simulink model "npc_system"  (R2022a)
settings: Solver=FixedStepDiscrete  StartTime=0.0  StopTime=1  FixedStep=step_size  RelTol=1e-3  EnableMultiTasking=on
values from neighbouring files (symbols this model uses):
  P = 11000.0    [param.sldd]
  step_size = 1.0E-7    [param.sldd]
  Tsw = 1.5E-5    [param.sldd]
undefined symbols (not defined in the file or in its folder): D1, DiscIntNeverNeededParam
libraries: simulink x14, eeGeneralControl x3, simulink_extras x1, spsEdgeDetectorLib x1, spsSampleandHoldLib x1
settings Model: DataDictionary=param.sldd  ExtModeTrigDuration=8  Creator=sgcesuser3  LastModifiedBy=sgcesuser3
settings SolverCC: AlgebraicLoopSolver=TrustRegion  AutoInsertRateTranBlk=on
settings DataIOCC: SaveOutput=off  SignalLogging=off  DSMLogging=off  SaveTime=off  ReturnWorkspaceOutputs=off
settings OptimizationCC: EnhancedBackFolding=on  PassReuseOutputArgsAs=Individual arguments  MaxStackSize=1024  OptimizeBlockOrder=speed  DifferentSizesBufferReuse=on  OptimizationCustomize=off  EfficientTunableParamExpr=on
settings DebuggingCC: ParameterTunabilityLossMsg=error  UnconnectedInputMsg=warning  UnconnectedOutputMsg=warning  UnconnectedLineMsg=warning  SFMachineParentedDataDiag=warning
settings HardwareCC: ProdBitPerChar=16  ProdBitPerInt=16  ProdBitPerPointer=32  ProdBitPerSizeT=32  ProdBitPerPtrDiffT=32  ProdLargestAtomicInteger=Integer  ProdLargestAtomicFloat=None  ProdWordSize=16  ProdLongLongMode=on  ProdHWDeviceType=Texas Instruments->C2000
settings ModelReferenceCC: PropagateSignalLabelsOutOfModel=off
settings SFSimCC: MATLABDynamicMemAlloc=off
settings RTWCC: SystemTargetFile=ert.tlc  HardwareBoard=TI Delfino F2837xS  TemplateMakefile=ert_default_tmf  Toolchain=Texas Instruments Code Composer Studio (C2000)  DLArmComputeVersion=19.05
settings CodeAppCC: ForceParamTrailComments=on  IgnoreCustomStorageClasses=off  OperatorAnnotations=on  SimulinkDataObjDesc=on  SFDataObjDesc=on  InsertBlockDesc=on
settings ERTTargetCC: CodeReplacementLibrary=TI C28x  ExtModeTransport=4  ExtModeStaticAlloc=on  ExtModeStaticAllocSize=5000  ExtModeMexFile=ext_xcp  ExtModeIntrfLevel=Level2 - Open

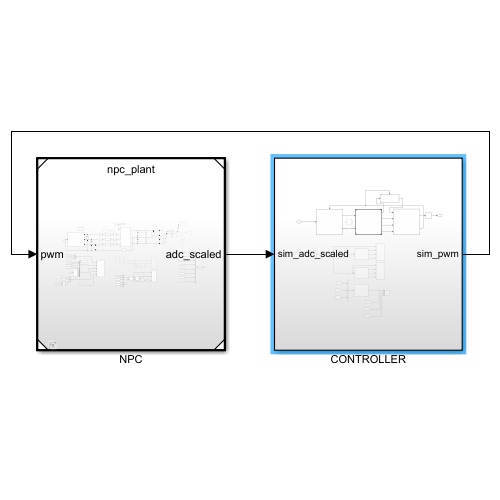
[thumbnail: Simulink's stored preview of the top-level diagram]
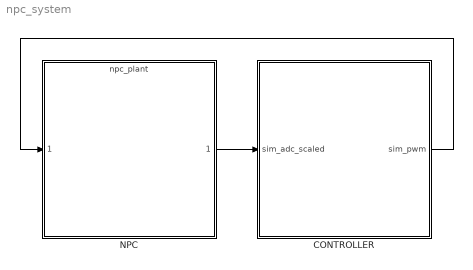
== system npc_system ==
  CONTROLLER : Subsystem
  NPC : ModelReference  ModelNameDialog=npc_plant.slx  SimulationMode=Normal  ModelReferenceVersion=4.130
  wires:
  CONTROLLER/1(sim_pwm) -> NPC/1
  NPC/1 -> CONTROLLER/1(sim_adc_scaled)

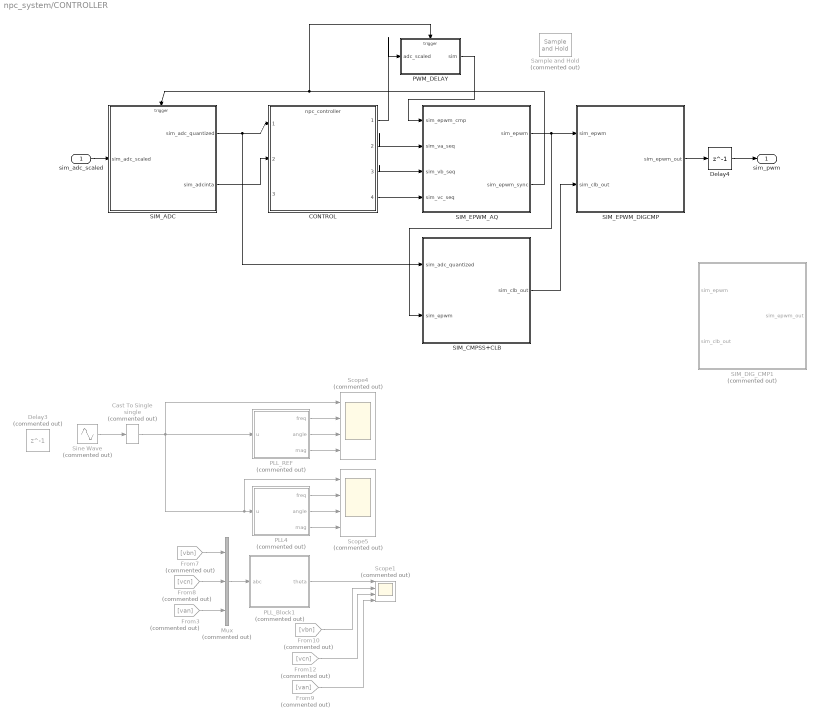
== system npc_system/CONTROLLER ==
  sim_adc_scaled : Inport
  CONTROL : ModelReference  ModelNameDialog=npc_controller.slx  SimulationMode=Normal  ScheduleRates=on  ModelEventPortInfo=P:D1[-2][0][0]  ModelReferenceVersion=4.1730
  Cast To Single : DataTypeConversion  Commented=on  OutDataTypeStr=single  SaturateOnIntegerOverflow=off  RndMeth=Floor
  Delay3 : Delay  Commented=on  DelayLength=1  InitialCondition=0
  Delay4 : Delay  DelayLength=1  InitialCondition=0
  From10 : From  Commented=on  GotoTag=vbn
  From12 : From  Commented=on  GotoTag=vcn
  From3 : From  Commented=on  GotoTag=van
  From7 : From  Commented=on  GotoTag=vbn
  From8 : From  Commented=on  GotoTag=vcn
  From9 : From  Commented=on  GotoTag=van
  Mux : Mux  Commented=on  Inputs=3
  PLL4 : Subsystem  Commented=on
  PLL_Block1 : Subsystem  Commented=on  TreatAsAtomicUnit=on
      settings: RTWFcnNameOpts=Use subsystem name
  PLL_REF : Subsystem  Commented=on
  PWM_DELAY : Subsystem  TreatAsAtomicUnit=on
  SIM_ADC : Subsystem  TreatAsAtomicUnit=on
  SIM_CMPSS+CLB : Subsystem
  SIM_DIG_CMP1 : Subsystem  Commented=on
  SIM_EPWM_AQ : Subsystem
  SIM_EPWM_DIGCMP : Subsystem
  Sample and Hold : spsSampleandHoldLib/Sample and Hold  Commented=on  ic=0  Ts=0
      settings: SourceProductBaseCode=PS
  Scope1 : Scope  Commented=on  NumInputPorts=4
  Scope4 : Scope  Commented=on  NumInputPorts=4
  Scope5 : Scope  Commented=on  NumInputPorts=4
  Sine Wave : Sin  Commented=on  Amplitude=220  Bias=100  Frequency=50*6.28
  sim_pwm : Outport
  wires:
  SIM_EPWM_AQ/2(sim_epwm_sync) -> PWM_DELAY/Trigger, SIM_ADC/Trigger
  SIM_ADC/2(sim_adcinta) -> CONTROL/2
  SIM_ADC/1(sim_adc_quantized) -> SIM_CMPSS+CLB/1(sim_adc_quantized), CONTROL/1
  PWM_DELAY/1(sim) -> SIM_EPWM_AQ/1(sim_epwm_cmp)
  CONTROL/2 -> SIM_EPWM_AQ/2(sim_va_seq)
  CONTROL/3 -> SIM_EPWM_AQ/3(sim_vb_seq)
  CONTROL/4 -> SIM_EPWM_AQ/4(sim_vc_seq)
  PLL_REF/1(freq) -> Scope4/2
  PLL_REF/2(angle) -> Scope4/3
  PLL_REF/3(mag) -> Scope4/4
  Sine Wave/1 -> Cast To Single/1
  Cast To Single/1 -> Scope5/1, PLL4/1(u), Scope4/1, PLL_REF/1(u)
  PLL4/3(mag) -> Scope5/4
  PLL4/2(angle) -> Scope5/3
  PLL4/1(freq) -> Scope5/2
  From9/1 -> Scope1/4
  From7/1 -> Mux/1
  From10/1 -> Scope1/2
  From3/1 -> Mux/3
  From8/1 -> Mux/2
  PLL_Block1/1(theta) -> Scope1/1
  Mux/1 -> PLL_Block1/1(abc)
  From12/1 -> Scope1/3
  sim_adc_scaled/1 -> SIM_ADC/1(sim_adc_scaled)
  Delay4/1 -> sim_pwm/1
  CONTROL/1 -> PWM_DELAY/1(adc_scaled)
  SIM_EPWM_DIGCMP/1(sim_epwm_out) -> Delay4/1
  SIM_EPWM_AQ/1(sim_epwm) -> SIM_CMPSS+CLB/2(sim_epwm), SIM_EPWM_DIGCMP/1(sim_epwm)
  SIM_CMPSS+CLB/1(sim_clb_out) -> SIM_EPWM_DIGCMP/2(sim_clb_out)

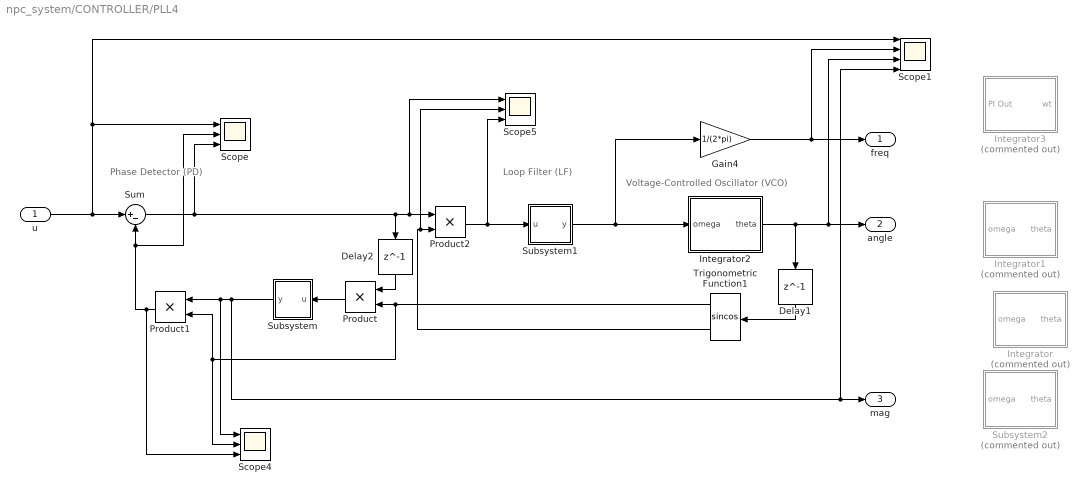
== system npc_system/CONTROLLER/PLL4 ==
  note: Voltage-Controlled Oscillator (VCO)
  note: Loop Filter (LF)
  note: Phase Detector (PD)
  u : Inport  OutDataTypeStr=single
  Delay1 : Delay  DelayLength=1
  Delay2 : Delay  DelayLength=1
  Gain4 : Gain  Gain=1/(2*pi)  ParamDataTypeStr=single  OutDataTypeStr=single
  Integrator : Subsystem  Commented=on
  Integrator1 : Subsystem  Commented=on
  Integrator2 : Subsystem
  Integrator3 : Subsystem  Commented=on
  Product : Product  OutDataTypeStr=single
  Product1 : Product  OutDataTypeStr=single
  Product2 : Product  OutDataTypeStr=single
  Scope : Scope  NumInputPorts=3
  Scope1 : Scope  NumInputPorts=4
  Scope4 : Scope  NumInputPorts=3
  Scope5 : Scope  NumInputPorts=3
  Subsystem : Subsystem
  Subsystem1 : Subsystem
  Subsystem2 : Subsystem  Commented=on
  Sum : Sum  Inputs=|+-  AccumDataTypeStr=single  OutDataTypeStr=single
  Trigonometric Function1 : Trigonometry  Operator=sincos
  freq : Outport  VectorParamsAs1DForOutWhenUnconnected=off
  angle : Outport  Port=2  VectorParamsAs1DForOutWhenUnconnected=off
  mag : Outport  Port=3  VectorParamsAs1DForOutWhenUnconnected=off
  wires:
  Gain4/1 -> Scope1/2, freq/1
  Integrator2/1(theta) -> Scope1/3, angle/1, Delay1/1
  Product2/1 -> Subsystem1/1(u), Scope5/3
  Sum/1 -> Scope/3, Product2/1, Scope5/1, Delay2/1
  Product1/1 -> Scope4/3, Scope/2, Sum/2
  Trigonometric Function1/1 -> Scope4/2, Product1/2, Product/2
  Product/1 -> Subsystem/1(u)
  Trigonometric Function1/2 -> Scope5/2, Product2/2
  u/1 -> Scope1/1, Scope/1, Sum/1
  Subsystem/1(y) -> Scope1/4, mag/1, Product1/1, Scope4/1
  Subsystem1/1(y) -> Gain4/1, Integrator2/1(omega)
  Delay1/1 -> Trigonometric Function1/1
  Delay2/1 -> Product/1

== system npc_system/CONTROLLER/PLL_Block1 ==
  abc : Inport
  Demux : Demux  Commented=on  Outputs=3
  If1 : If  Commented=on  IfExpression=(u1 > 0)  ShowElse=off
  SRF_PLL : Subsystem
  Subsystem : Subsystem  Commented=on
  theta : Outport  OutDataTypeStr=single
  wires:
  SRF_PLL/3(theta) -> theta/1
  Subsystem/1(Out1) -> If1/1
  abc/1 -> SRF_PLL/1(Vabc), Demux/1
  Demux/1 -> Subsystem/1(In1)

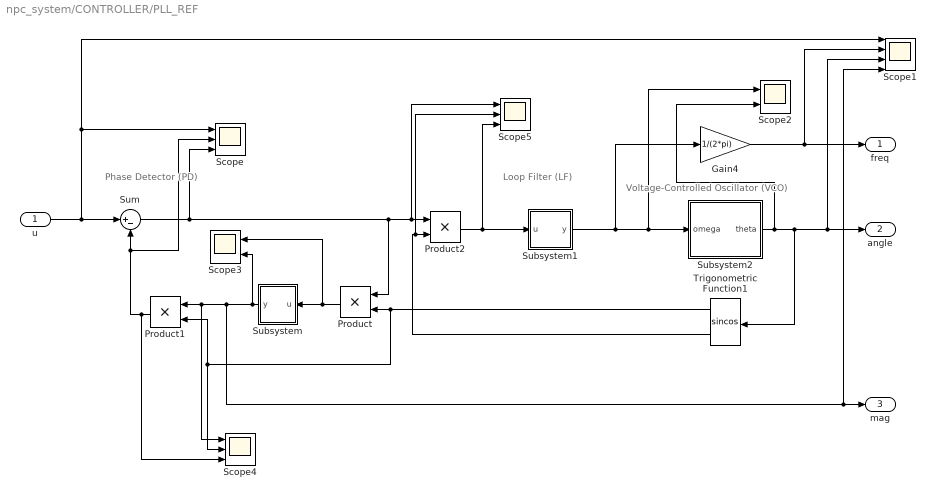
== system npc_system/CONTROLLER/PLL_REF ==
  note: Loop Filter (LF)
  note: Phase Detector (PD)
  note: Voltage-Controlled Oscillator (VCO)
  u : Inport  OutDataTypeStr=single
  Gain4 : Gain  Gain=1/(2*pi)  ParamDataTypeStr=single  OutDataTypeStr=single
  Product : Product  OutDataTypeStr=single
  Product1 : Product  OutDataTypeStr=single
  Product2 : Product  OutDataTypeStr=single
  Scope : Scope  NumInputPorts=3
  Scope1 : Scope  NumInputPorts=4
  Scope2 : Scope  NumInputPorts=2
  Scope3 : Scope  NumInputPorts=2
  Scope4 : Scope  NumInputPorts=3
  Scope5 : Scope  NumInputPorts=3
  Subsystem : Subsystem
  Subsystem1 : Subsystem
  Subsystem2 : Subsystem
  Sum : Sum  Inputs=|+-  AccumDataTypeStr=single  OutDataTypeStr=single
  Trigonometric Function1 : Trigonometry  Operator=sincos
  freq : Outport  VectorParamsAs1DForOutWhenUnconnected=off
  angle : Outport  Port=2  VectorParamsAs1DForOutWhenUnconnected=off
  mag : Outport  Port=3  VectorParamsAs1DForOutWhenUnconnected=off
  wires:
  Subsystem1/1(y) -> Scope2/1, Subsystem2/1(omega), Gain4/1
  Subsystem2/1(theta) -> Scope2/2, Trigonometric Function1/1, Scope1/3, angle/1
  Subsystem/1(y) -> Scope3/2, Scope1/4, mag/1, Scope4/1, Product1/1
  Trigonometric Function1/1 -> Scope4/2, Product1/2, Product/2
  Trigonometric Function1/2 -> Scope5/2, Product2/2
  Sum/1 -> Scope/3, Product/1, Scope5/1, Product2/1
  Gain4/1 -> Scope1/2, freq/1
  u/1 -> Scope1/1, Scope/1, Sum/1
  Product/1 -> Scope3/1, Subsystem/1(u)
  Product1/1 -> Scope4/3, Scope/2, Sum/2
  Product2/1 -> Scope5/3, Subsystem1/1(u)

== system npc_system/CONTROLLER/PWM_DELAY ==
  adc_scaled : Inport
  Trigger : TriggerPort  VariantControl=Variant  PortDimensions=1
  sim : Outport
  wires:
  adc_scaled/1 -> sim/1

== system npc_system/CONTROLLER/SIM_ADC ==
  sim_adc_scaled : Inport
  Trigger : TriggerPort  TriggerType=falling  VariantControl=Variant  PortDimensions=1
  Cast To Single : DataTypeConversion  OutDataTypeStr=single  SaturateOnIntegerOverflow=off  RndMeth=Floor
  Chart2 : Stateflow chart  TreatAsAtomicUnit=on
  Idealized ADC quantizer1 : simulink_extras/Additional Discrete/Idealized ADC quantizer  NumberOfConverterBits=12  Vmin=0  Vmax=3.3  OutputDataType=double  OutputNegativeValues=off
  Zero-Order Hold : ZeroOrderHold  SampleTime=-1
  sim_adc_quantized : Outport
  sim_adcinta : Outport  Port=2
  wires:
  Zero-Order Hold/1 -> Idealized ADC quantizer1/1
  sim_adc_scaled/1 -> Zero-Order Hold/1
  Idealized ADC quantizer1/1 -> Cast To Single/1
  Chart2/1(adcinta()) -> sim_adcinta/1
  Cast To Single/1 -> sim_adc_quantized/1

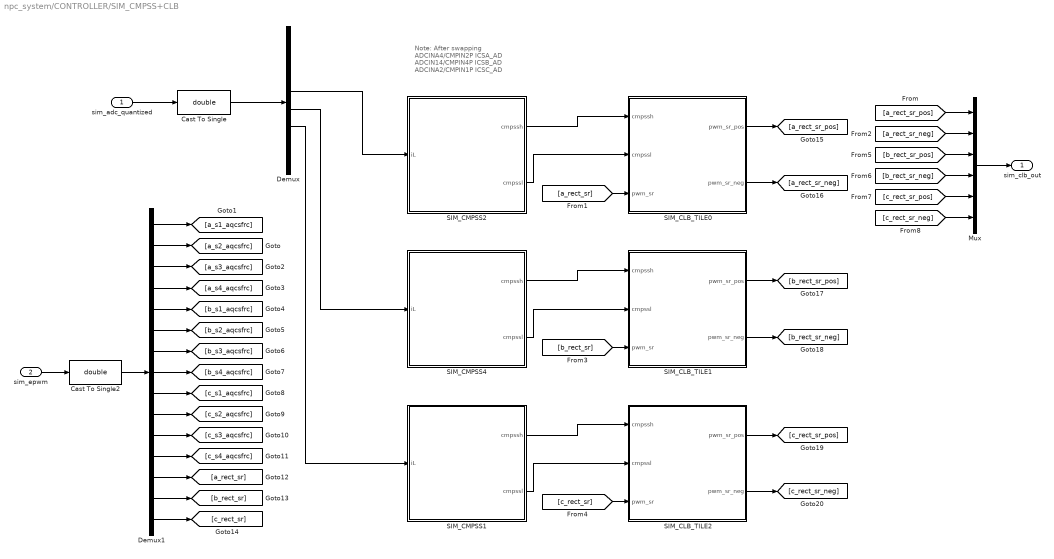
== system npc_system/CONTROLLER/SIM_CMPSS+CLB ==
  note: Note: After swapping
      | ADCINA4/CMPIN2P ICSA_AD
      | ADCIN14/CMPIN4P ICSB_AD
      | ADCINA2/CMPIN1P ICSC_AD
  sim_adc_quantized : Inport
  sim_epwm : Inport  Port=2
  Cast To Single : DataTypeConversion  OutDataTypeStr=double  SaturateOnIntegerOverflow=off  RndMeth=Floor
  Cast To Single2 : DataTypeConversion  OutDataTypeStr=double  SaturateOnIntegerOverflow=off  RndMeth=Floor
  Demux : Demux  Outputs=8
  Demux1 : Demux  Outputs=15
  Mux : Mux  Inputs=6
  SIM_CLB_TILE0 : Stateflow chart  TreatAsAtomicUnit=on
  SIM_CLB_TILE1 : Stateflow chart  TreatAsAtomicUnit=on
  SIM_CLB_TILE2 : Stateflow chart  TreatAsAtomicUnit=on
  SIM_CMPSS1 : Stateflow chart  TreatAsAtomicUnit=on
  SIM_CMPSS2 : Stateflow chart  TreatAsAtomicUnit=on
  SIM_CMPSS4 : Stateflow chart  TreatAsAtomicUnit=on
  sim_clb_out : Outport
  wires:
  Mux/1 -> sim_clb_out/1
  Demux1/1 -> [a_s1_aqcsfrc]
  sim_epwm/1 -> Cast To Single2/1
  sim_adc_quantized/1 -> Cast To Single/1
  Demux/4 -> SIM_CMPSS2/1(iL)
  Demux1/2 -> [a_s2_aqcsfrc]
  Demux1/3 -> [a_s3_aqcsfrc]
  Demux1/4 -> [a_s4_aqcsfrc]
  Demux1/5 -> [b_s1_aqcsfrc]
  Demux1/6 -> [b_s2_aqcsfrc]
  Demux1/7 -> [b_s3_aqcsfrc]
  Demux1/8 -> [b_s4_aqcsfrc]
  Demux1/9 -> [c_s1_aqcsfrc]
  Demux1/10 -> [c_s2_aqcsfrc]
  Demux1/11 -> [c_s3_aqcsfrc]
  Demux1/12 -> [c_s4_aqcsfrc]
  Cast To Single/1 -> Demux/1
  Cast To Single2/1 -> Demux1/1
  [a_rect_sr] -> SIM_CLB_TILE0/3(pwm_sr)
  SIM_CLB_TILE0/1(pwm_sr_pos) -> [a_rect_sr_pos]
  SIM_CLB_TILE0/2(pwm_sr_neg) -> [a_rect_sr_neg]
  Demux1/13 -> [a_rect_sr]
  Demux1/14 -> [b_rect_sr]
  Demux1/15 -> [c_rect_sr]
  [a_rect_sr_neg] -> Mux/2
  [a_rect_sr_pos] -> Mux/1
  [b_rect_sr] -> SIM_CLB_TILE1/3(pwm_sr)
  [c_rect_sr] -> SIM_CLB_TILE2/3(pwm_sr)
  SIM_CMPSS4/1(cmpssh) -> SIM_CLB_TILE1/1(cmpssh)
  SIM_CMPSS4/2(cmpssl) -> SIM_CLB_TILE1/2(cmpssl)
  SIM_CMPSS1/1(cmpssh) -> SIM_CLB_TILE2/1(cmpssh)
  SIM_CMPSS1/2(cmpssl) -> SIM_CLB_TILE2/2(cmpssl)
  SIM_CMPSS2/1(cmpssh) -> SIM_CLB_TILE0/1(cmpssh)
  SIM_CMPSS2/2(cmpssl) -> SIM_CLB_TILE0/2(cmpssl)
  Demux/5 -> SIM_CMPSS4/1(iL)
  Demux/6 -> SIM_CMPSS1/1(iL)
  SIM_CLB_TILE1/1(pwm_sr_pos) -> [b_rect_sr_pos]
  SIM_CLB_TILE1/2(pwm_sr_neg) -> [b_rect_sr_neg]
  SIM_CLB_TILE2/1(pwm_sr_pos) -> [c_rect_sr_pos]
  SIM_CLB_TILE2/2(pwm_sr_neg) -> [c_rect_sr_neg]
  [c_rect_sr_neg] -> Mux/6
  [c_rect_sr_pos] -> Mux/5
  [b_rect_sr_neg] -> Mux/4
  [b_rect_sr_pos] -> Mux/3

== system npc_system/CONTROLLER/SIM_DIG_CMP1 ==
  sim_epwm : Inport
  sim_clb_out : Inport  Port=2
  Demux : Demux  Outputs=12
  Demux1 : Demux  Outputs=6
  Mux : Mux  Inputs=12
  sim_epwm_out : Outport
  wires:
  Demux1/6 -> Mux/12  "C_S4"
  Demux1/5 -> Mux/9  "C_S1"
  Demux1/4 -> Mux/8  "B_S4"
  Demux1/3 -> Mux/5  "B_S1"
  Demux1/2 -> Mux/4  "A_S4"
  Demux1/1 -> Mux/1  "A_S1"
  sim_clb_out/1 -> Demux1/1
  Demux/11 -> Mux/11  "C_S3"
  Demux/10 -> Mux/10  "C_S2"
  Demux/7 -> Mux/7  "B_S3"
  Demux/6 -> Mux/6  "B_S2"
  Demux/3 -> Mux/3  "A_S3"
  Demux/2 -> Mux/2  "A_S2"
  sim_epwm/1 -> Demux/1
  Mux/1 -> sim_epwm_out/1

== system npc_system/CONTROLLER/SIM_EPWM_AQ ==
  sim_epwm_cmp : Inport
  sim_va_seq : Inport  Port=2
  sim_vb_seq : Inport  Port=3
  sim_vc_seq : Inport  Port=4
  sim_carrier : simulink/Sources/Repeating Sequence Interpolated  OutValues=[0 1538 0].'  TimeValues=[0 Tsw/2 Tsw].'  LookUpMeth=Interpolation-Use End Values  tsamp=step_size  OutMin=[]  OutMax=[]  OutDataTypeStr=double  OutputDataTypeScalingMode=double  OutDataType=fixdt(0,8)  OutScaling=2^-10
  sim_epwm. : Subsystem  Variant=on
  sim_epwm : Outport
  sim_epwm_sync : Outport  Port=2
  wires:
  sim_epwm_cmp/1 -> sim_epwm./1(sim_epwm_cmp)
  sim_epwm./1(sim_epwm) -> sim_epwm/1
  sim_carrier/1 -> sim_epwm./2(sim_carrier)
  sim_epwm./2(pwm_sync) -> sim_epwm_sync/1
  sim_va_seq/1 -> sim_epwm./3(sim_va_seq)
  sim_vb_seq/1 -> sim_epwm./4(sim_vb_seq)
  sim_vc_seq/1 -> sim_epwm./5(sim_vc_seq)

== system npc_system/CONTROLLER/SIM_EPWM_DIGCMP ==
  sim_epwm : Inport
  sim_clb_out : Inport  Port=2
  Demux : Demux  Outputs=15
  Demux1 : Demux  Outputs=6
  Mux : Mux  Inputs=12
  sim_epwm_out : Outport
  wires:
  Mux/1 -> sim_epwm_out/1
  sim_epwm/1 -> Demux/1
  Demux/2 -> Mux/2  "A_S2"
  Demux/3 -> Mux/3  "A_S3"
  sim_clb_out/1 -> Demux1/1
  Demux/6 -> Mux/6  "B_S2"
  Demux/7 -> Mux/7  "B_S3"
  Demux/10 -> Mux/10  "C_S2"
  Demux/11 -> Mux/11  "C_S3"
  Demux1/1 -> Mux/1  "A_S1"
  Demux1/2 -> Mux/4  "A_S4"
  Demux1/3 -> Mux/5  "B_S1"
  Demux1/4 -> Mux/8  "B_S4"
  Demux1/5 -> Mux/9  "C_S1"
  Demux1/6 -> Mux/12  "C_S4"

== system npc_system/CONTROLLER/PLL4/Integrator ==
  omega : Inport  OutDataTypeStr=single
  Integrator with Wrapped State (Discrete or Continuous) : eeGeneralControl/Integrator with Wrapped State (Discrete or Continuous)  LabelModeActiveChoice=Discrete  WrappedStateUpperValue=2*pi  WrappedStateLowerValue=0  x0=0  Ts=-1
      settings: SourceProductBaseCode=PS
  theta : Outport
  wires:
  Integrator with Wrapped State (Discrete or Continuous)/1 -> theta/1
  omega/1 -> Integrator with Wrapped State (Discrete or Continuous)/1

== system npc_system/CONTROLLER/PLL4/Integrator1 ==
  omega : Inport  OutDataTypeStr=single
  Accumulation : Subsystem  TreatAsAtomicUnit=on
  Compare To Constant : simulink/Logic and Bit Operations/Compare To Constant  relop=>=  const=2*pi  OutDataTypeStr=boolean
  If : If  IfExpression=u1
  Merge : Merge
  Reset Integrator : Subsystem  TreatAsAtomicUnit=on
  Unit Delay : UnitDelay  SampleTime=-1  HasFrameUpgradeWarning=on
  theta : Outport
  wires:
  omega/1 -> Compare To Constant/1, Accumulation/1(In1)
  Compare To Constant/1 -> If/1
  If/1 -> Reset Integrator/Action
  If/2 -> Accumulation/Action
  Reset Integrator/1(Out) -> Merge/1
  Accumulation/1(Out) -> Merge/2
  Merge/1 -> Unit Delay/1
  Unit Delay/1 -> theta/1

== system npc_system/CONTROLLER/PLL4/Integrator2 ==
  omega : Inport  OutDataTypeStr=single
  Compare To Constant2 : simulink/Logic and Bit Operations/Compare To Constant  relop=>=  const=2*pi  OutDataTypeStr=boolean
  Constant : Constant  Commented=on  Value=313  OutDataTypeStr=single
  Delay1 : Delay  DelayLength=1  InitialCondition=0
  Delay2 : Delay  DelayLength=1  InitialCondition=0  ExternalReset=Level
      settings: InputPortMap=u0,r5
  Product : Product  OutDataTypeStr=single
  Scope2 : Scope  NumInputPorts=3
  Sum : Sum  Inputs=|++  AccumDataTypeStr=single  OutDataTypeStr=single
  Ts : Constant  Value=step_size  OutDataTypeStr=single
  theta : Outport
  wires:
  Sum/1 -> Delay2/1, Scope2/3, theta/1
  Product/1 -> Sum/1, Scope2/1
  Ts/1 -> Product/2
  Delay2/1 -> Scope2/2, Delay1/1, Sum/2
  Delay1/1 -> Compare To Constant2/1
  Compare To Constant2/1 -> Delay2/2
  omega/1 -> Product/1

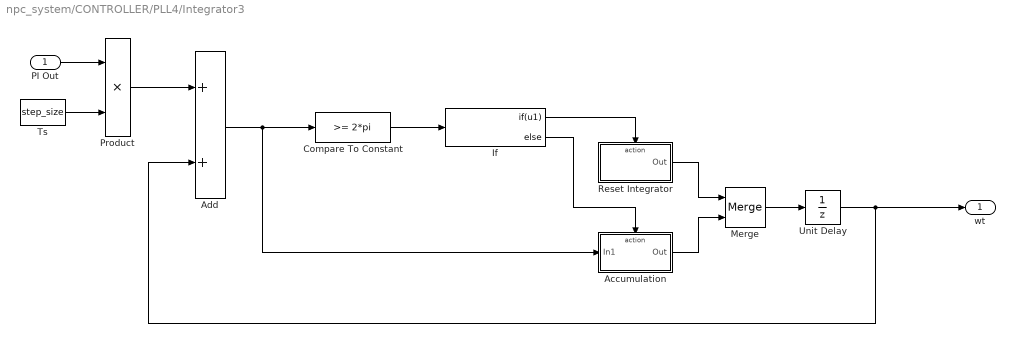
== system npc_system/CONTROLLER/PLL4/Integrator3 ==
  PI Out : Inport  OutDataTypeStr=single
  Accumulation : Subsystem  TreatAsAtomicUnit=on
  Add : Sum  AccumDataTypeStr=single
  Compare To Constant : simulink/Logic and Bit Operations/Compare To Constant  relop=>=  const=2*pi  OutDataTypeStr=boolean
  If : If  IfExpression=u1
  Merge : Merge
  Product : Product  OutDataTypeStr=single
  Reset Integrator : Subsystem  TreatAsAtomicUnit=on
  Ts : Constant  Value=step_size  OutDataTypeStr=single
  Unit Delay : UnitDelay  SampleTime=-1  HasFrameUpgradeWarning=on
  wt : Outport
  wires:
  PI Out/1 -> Product/1
  Ts/1 -> Product/2
  Product/1 -> Add/1
  Add/1 -> Accumulation/1(In1), Compare To Constant/1
  Compare To Constant/1 -> If/1
  If/1 -> Reset Integrator/Action
  If/2 -> Accumulation/Action
  Reset Integrator/1(Out) -> Merge/1
  Accumulation/1(Out) -> Merge/2
  Merge/1 -> Unit Delay/1
  Unit Delay/1 -> wt/1, Add/2

== system npc_system/CONTROLLER/PLL4/Subsystem ==
  u : Inport
  Constant1 : Constant  OutDataTypeStr=single  SampleTime=-1
  Delay3 : Delay  DelayLength=1  InitialConditionSource=Input port  InitialCondition=0
      settings: InputPortMap=u0,p4
  Gain1 : Gain  Gain=1000  ParamDataTypeStr=single  OutDataTypeStr=single
  Product : Product  OutDataTypeStr=single
  Scope2 : Scope  NumInputPorts=3
  Sum : Sum  Inputs=|++  AccumDataTypeStr=single  OutDataTypeStr=single
  Ts : Constant  Value=step_size  OutDataTypeStr=single
  y : Outport  VectorParamsAs1DForOutWhenUnconnected=off
  wires:
  u/1 -> Gain1/1
  Sum/1 -> Delay3/1, y/1, Scope2/3
  Delay3/1 -> Scope2/2, Sum/2
  Ts/1 -> Product/2
  Product/1 -> Scope2/1, Sum/1
  Gain1/1 -> Product/1
  Constant1/1 -> Delay3/2

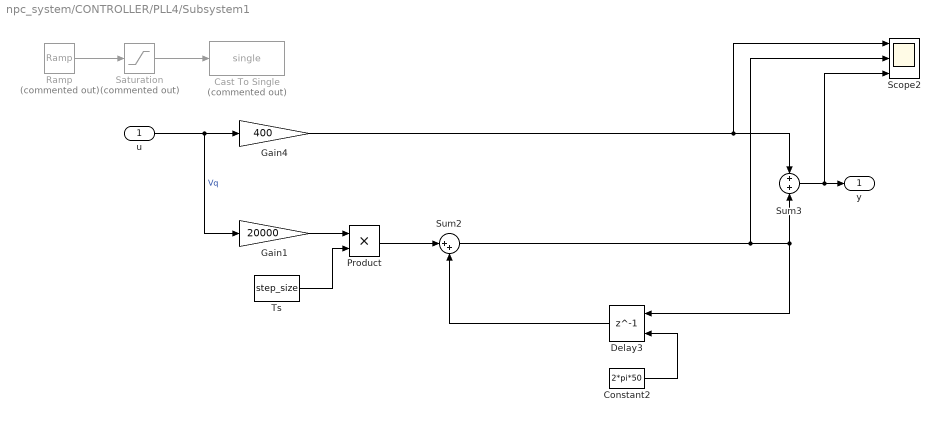
== system npc_system/CONTROLLER/PLL4/Subsystem1 ==
  u : Inport
  Cast To Single : DataTypeConversion  Commented=on  OutDataTypeStr=single  SaturateOnIntegerOverflow=off  RndMeth=Floor
  Constant2 : Constant  Value=2*pi*50  OutDataTypeStr=single  SampleTime=-1
  Delay3 : Delay  DelayLength=1  InitialConditionSource=Input port  InitialCondition=0
      settings: InputPortMap=u0,p4
  Gain1 : Gain  Gain=20000  ParamDataTypeStr=single  OutDataTypeStr=single
  Gain4 : Gain  Gain=400  ParamDataTypeStr=single  OutDataTypeStr=single
  Product : Product  OutDataTypeStr=single
  Ramp : simulink/Sources/Ramp  Commented=on  slope=-100000  start=0  InitialOutput=1000
  Saturation : Saturate  Commented=on  UpperLimit=1000  LowerLimit=0
  Scope2 : Scope  NumInputPorts=3
  Sum2 : Sum  Inputs=|++  AccumDataTypeStr=single  OutDataTypeStr=single
  Sum3 : Sum  Inputs=+|+  AccumDataTypeStr=single  OutDataTypeStr=single
  Ts : Constant  Value=step_size  OutDataTypeStr=single
  y : Outport  VectorParamsAs1DForOutWhenUnconnected=off
  wires:
  u/1 -> Gain1/1, Gain4/1  "Vq"
  Sum3/1 -> Scope2/3, y/1
  Product/1 -> Sum2/1
  Ts/1 -> Product/2
  Delay3/1 -> Sum2/2
  Gain1/1 -> Product/1
  Sum2/1 -> Scope2/2, Delay3/1, Sum3/2
  Constant2/1 -> Delay3/2
  Gain4/1 -> Scope2/1, Sum3/1
  Ramp/1 -> Saturation/1
  Saturation/1 -> Cast To Single/1

== system npc_system/CONTROLLER/PLL4/Subsystem2 ==
  omega : Inport
  Compare To Constant : simulink/Logic and Bit Operations/Compare To Constant  relop=<  const=0  OutDataTypeStr=boolean
  Compare To Constant1 : simulink/Logic and Bit Operations/Compare To Constant  relop=>=  const=2*pi  OutDataTypeStr=boolean
  Initial : InitialCondition  Value=0
  Integrator : DiscreteIntegrator  ExternalReset=sampled level  InitialConditionSource=external  SampleTime=-1  ShowStatePort=on  ICPrevOutput=DiscIntNeverNeededParam  ICPrevScaledInput=DiscIntNeverNeededParam
  Logical Operator : Logic  Operator=OR  AllPortsSameDT=off  OutDataTypeStr=boolean
  Subsystem : Subsystem
  theta : Outport
  wires:
  Subsystem/1(y) -> Initial/1
  Compare To Constant1/1 -> Logical Operator/2
  Integrator/1 -> theta/1
  Compare To Constant/1 -> Logical Operator/1
  Logical Operator/1 -> Integrator/2
  omega/1 -> Integrator/1
  Initial/1 -> Integrator/3
  Integrator/State -> Compare To Constant1/1, Subsystem/1(u1), Compare To Constant/1

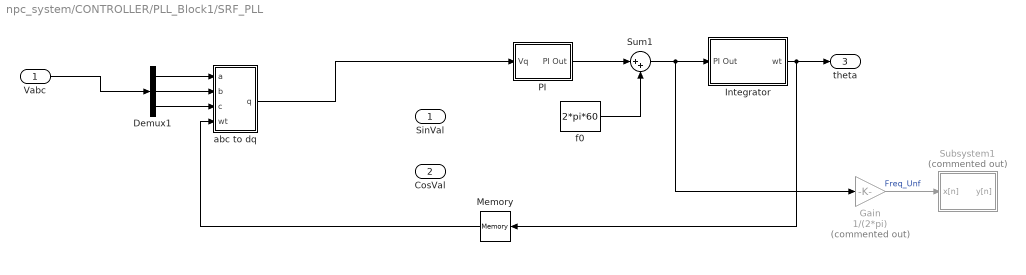
== system npc_system/CONTROLLER/PLL_Block1/SRF_PLL ==
  Vabc : Inport
  Demux1 : Demux  Outputs=3
  Gain : Gain  Commented=on  Gain=1/(2*pi)
  Integrator : Subsystem
  Memory : Memory  InheritSampleTime=on  LinearizeAsDelay=on
  PI : Subsystem
  Subsystem1 : Subsystem  Commented=on
  Sum1 : Sum  Inputs=|++  AccumDataTypeStr=single  OutDataTypeStr=single
  abc to dq : Subsystem
  f0 : Constant  Value=2*pi*60  OutDataTypeStr=fixdt('single', 'DataTypeOverride', 'Off')
  SinVal : Outport  VectorParamsAs1DForOutWhenUnconnected=off
  CosVal : Outport  Port=2  VectorParamsAs1DForOutWhenUnconnected=off
  theta : Outport  Port=3  OutDataTypeStr=single  VectorParamsAs1DForOutWhenUnconnected=off
  wires:
  Vabc/1 -> Demux1/1
  Memory/1 -> abc to dq/4(wt)
  Integrator/1(wt) -> Memory/1, theta/1
  abc to dq/1(q) -> PI/1(Vq)
  f0/1 -> Sum1/2
  Gain/1 -> Subsystem1/1(x[n])  "Freq_Unf"
  PI/1(PI Out) -> Sum1/1
  Sum1/1 -> Gain/1, Integrator/1(PI Out)
  Demux1/1 -> abc to dq/1(a)
  Demux1/2 -> abc to dq/2(b)
  Demux1/3 -> abc to dq/3(c)

== system npc_system/CONTROLLER/PLL_Block1/Subsystem ==
  In1 : Inport
  Cast To Single : DataTypeConversion  OutDataTypeStr=single  SaturateOnIntegerOverflow=off  RndMeth=Floor
  Constant2 : Constant  Value=0
  GreaterThan1 : RelationalOperator  Operator=>  OutDataTypeStr=boolean  RndMeth=Simplest  InputSameDT=off
  Initialize at Zero Crossing : Subsystem  TreatAsAtomicUnit=on
  Out1 : Outport
  wires:
  GreaterThan1/1 -> Initialize at Zero Crossing/Trigger, Initialize at Zero Crossing/1(In1)
  Constant2/1 -> GreaterThan1/2
  Initialize at Zero Crossing/1(Out1) -> Cast To Single/1
  In1/1 -> GreaterThan1/1
  Cast To Single/1 -> Out1/1

== system npc_system/CONTROLLER/PLL_REF/Subsystem ==
  u : Inport
  Constant : Constant  OutDataTypeStr=single  SampleTime=-1
  Constant1 : Constant  Value=0  OutDataTypeStr=single  SampleTime=-1
  Data Type Conversion Inherited : simulink/Signal Attributes/Data Type Conversion Inherited  ConvertRealWorld=Real World Value  DoSatur=off
      settings: SourceProductBaseCode=SL
  Gain : Gain  Gain=1000  ParamDataTypeStr=single  OutDataTypeStr=single
  Integrator (Discrete or Continuous) : eeGeneralControl/Integrator (Discrete or Continuous)  LabelModeActiveChoice=Discrete  ExternalReset=rising  LimitType=Anti-windup  B=inf  A=-inf  Ts=-1
      settings: SourceProductBaseCode=PS
  y : Outport  VectorParamsAs1DForOutWhenUnconnected=off
  wires:
  Data Type Conversion Inherited/1 -> Integrator (Discrete or Continuous)/3
  Gain/1 -> Integrator (Discrete or Continuous)/1
  u/1 -> Gain/1, Data Type Conversion Inherited/1
  Integrator (Discrete or Continuous)/1 -> y/1
  Constant1/1 -> Integrator (Discrete or Continuous)/2
  Constant/1 -> Data Type Conversion Inherited/2

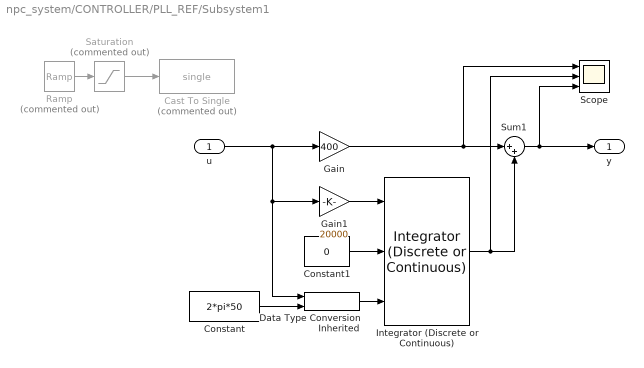
== system npc_system/CONTROLLER/PLL_REF/Subsystem1 ==
  u : Inport
  Cast To Single : DataTypeConversion  Commented=on  OutDataTypeStr=single  SaturateOnIntegerOverflow=off  RndMeth=Floor
  Constant : Constant  Value=2*pi*50  OutDataTypeStr=single  SampleTime=-1
  Constant1 : Constant  Value=0  OutDataTypeStr=single  SampleTime=-1
  Data Type Conversion Inherited : simulink/Signal Attributes/Data Type Conversion Inherited  ConvertRealWorld=Real World Value  DoSatur=off
      settings: SourceProductBaseCode=SL
  Gain : Gain  Gain=400  ParamDataTypeStr=single  OutDataTypeStr=single
  Gain1 : Gain  Gain=20000  ParamDataTypeStr=single  OutDataTypeStr=single
  Integrator (Discrete or Continuous) : eeGeneralControl/Integrator (Discrete or Continuous)  LabelModeActiveChoice=Discrete  ExternalReset=level  LimitType=Anti-windup  B=inf  A=-inf  Ts=-1
      settings: SourceProductBaseCode=PS
  Ramp : simulink/Sources/Ramp  Commented=on  slope=-1000  start=0  InitialOutput=100
  Saturation : Saturate  Commented=on  UpperLimit=100  LowerLimit=0
  Scope : Scope  NumInputPorts=3
  Sum1 : Sum  Inputs=|++  AccumDataTypeStr=single  OutDataTypeStr=single
  y : Outport  VectorParamsAs1DForOutWhenUnconnected=off
  wires:
  Data Type Conversion Inherited/1 -> Integrator (Discrete or Continuous)/3
  Gain/1 -> Scope/1, Sum1/1
  u/1 -> Gain/1, Gain1/1, Data Type Conversion Inherited/1
  Gain1/1 -> Integrator (Discrete or Continuous)/1
  Constant1/1 -> Integrator (Discrete or Continuous)/2
  Constant/1 -> Data Type Conversion Inherited/2
  Sum1/1 -> Scope/3, y/1
  Integrator (Discrete or Continuous)/1 -> Scope/2, Sum1/2
  Saturation/1 -> Cast To Single/1
  Ramp/1 -> Saturation/1

== system npc_system/CONTROLLER/PLL_REF/Subsystem2 ==
  omega : Inport
  Compare To Constant : simulink/Logic and Bit Operations/Compare To Constant  relop=<  const=0  OutDataTypeStr=boolean
  Compare To Constant1 : simulink/Logic and Bit Operations/Compare To Constant  relop=>=  const=2*pi  OutDataTypeStr=boolean
  Initial : InitialCondition  Value=0
  Integrator : DiscreteIntegrator  ExternalReset=sampled level  InitialConditionSource=external  SampleTime=-1  ShowStatePort=on  ICPrevOutput=DiscIntNeverNeededParam  ICPrevScaledInput=DiscIntNeverNeededParam
  Logical Operator : Logic  Operator=OR  AllPortsSameDT=off  OutDataTypeStr=boolean
  Subsystem : Subsystem
  theta : Outport
  wires:
  Integrator/State -> Compare To Constant/1, Subsystem/1(u1), Compare To Constant1/1
  Initial/1 -> Integrator/3
  omega/1 -> Integrator/1
  Logical Operator/1 -> Integrator/2
  Compare To Constant/1 -> Logical Operator/1
  Integrator/1 -> theta/1
  Compare To Constant1/1 -> Logical Operator/2
  Subsystem/1(y) -> Initial/1

== system npc_system/CONTROLLER/SIM_EPWM_AQ/sim_epwm. ==
  note: 1) Add Subsystem or Model blocks as valid variant choices.
      | 2) You cannot connect blocks at this level. At simulation, connectivity is automatically
      | determined, based on the active variant and port name matching.
  sim_epwm_cmp : Inport
  sim_carrier : Inport  Port=2
  sim_va_seq : Inport  Port=3
  sim_vb_seq : Inport  Port=4
  sim_vc_seq : Inport  Port=5
  codegen : Subsystem  VariantControl=sim_en==false
  sim : Subsystem  VariantControl=sim_en==true
  sim_epwm : Outport
  pwm_sync : Outport  Port=2

== system npc_system/CONTROLLER/PLL4/Integrator1/Accumulation ==
  In1 : Inport  OutDataTypeStr=single
  Action Port : ActionPort
  Out : Outport  OutDataTypeStr=single
  wires:
  In1/1 -> Out/1

== system npc_system/CONTROLLER/PLL4/Integrator1/Reset Integrator ==
  Action Port : ActionPort
  Constant1 : Constant  Value=0  OutDataTypeStr=single  SampleTime=-1
  Out : Outport
  wires:
  Constant1/1 -> Out/1

== system npc_system/CONTROLLER/PLL4/Integrator3/Accumulation ==
  In1 : Inport  OutDataTypeStr=single
  Action Port : ActionPort
  Out : Outport  OutDataTypeStr=single
  wires:
  In1/1 -> Out/1

== system npc_system/CONTROLLER/PLL4/Integrator3/Reset Integrator ==
  Action Port : ActionPort
  Constant1 : Constant  Value=0  OutDataTypeStr=single
  Out : Outport
  wires:
  Constant1/1 -> Out/1

== system npc_system/CONTROLLER/PLL4/Subsystem2/Subsystem ==
  u1 : Inport
  Bias : Bias  Bias=-0  SaturateOnIntegerOverflow=off
  Gain : Gain  Gain=1/(2*pi-0)
  Gain1 : Gain  Gain=(2*pi-0)
  Rounding Function : Rounding
  Sum1 : Sum  Inputs=|+-
  y : Outport  VectorParamsAs1DForOutWhenUnconnected=off
  wires:
  Rounding Function/1 -> Gain1/1
  u1/1 -> Sum1/1, Bias/1
  Gain/1 -> Rounding Function/1
  Sum1/1 -> y/1
  Bias/1 -> Gain/1
  Gain1/1 -> Sum1/2

== system npc_system/CONTROLLER/PLL_Block1/SRF_PLL/Integrator ==
  PI Out : Inport  OutDataTypeStr=single
  Accumulation : Subsystem  TreatAsAtomicUnit=on
  Add : Sum  AccumDataTypeStr=single
  Compare To Constant : simulink/Logic and Bit Operations/Compare To Constant  relop=>=  const=2*pi  OutDataTypeStr=boolean
  If : If  IfExpression=u1
  Merge : Merge
  Product : Product  OutDataTypeStr=single
  Reset Integrator : Subsystem  TreatAsAtomicUnit=on
  Ts : Constant  Value=Tsw  OutDataTypeStr=single
  Unit Delay : UnitDelay  SampleTime=-1  HasFrameUpgradeWarning=on
  wt : Outport
  wires:
  PI Out/1 -> Product/1
  Ts/1 -> Product/2
  Product/1 -> Add/1
  Add/1 -> Accumulation/1(In1), Compare To Constant/1
  Compare To Constant/1 -> If/1
  If/1 -> Reset Integrator/Action
  If/2 -> Accumulation/Action
  Reset Integrator/1(Out) -> Merge/1
  Accumulation/1(Out) -> Merge/2
  Merge/1 -> Unit Delay/1
  Unit Delay/1 -> wt/1, Add/2

== system npc_system/CONTROLLER/PLL_Block1/SRF_PLL/PI ==
  Vq : Inport
  Ki : Gain  Gain=200
  Kp : Gain  Gain=0.5
  Sum : Sum  Inputs=|++
  Sum1 : Sum  Inputs=+|+
  Ts/2 : Gain  Gain=Tsw/2
  Unit Delay : UnitDelay  SampleTime=-1  HasFrameUpgradeWarning=on
  PI Out : Outport
  wires:
  Ts/2/1 -> Sum/1
  Sum1/1 -> PI Out/1
  Ki/1 -> Ts/2/1
  Vq/1 -> Ki/1, Kp/1  "Vq"
  Unit Delay/1 -> Sum/2
  Kp/1 -> Sum1/1
  Sum/1 -> Sum1/2, Unit Delay/1

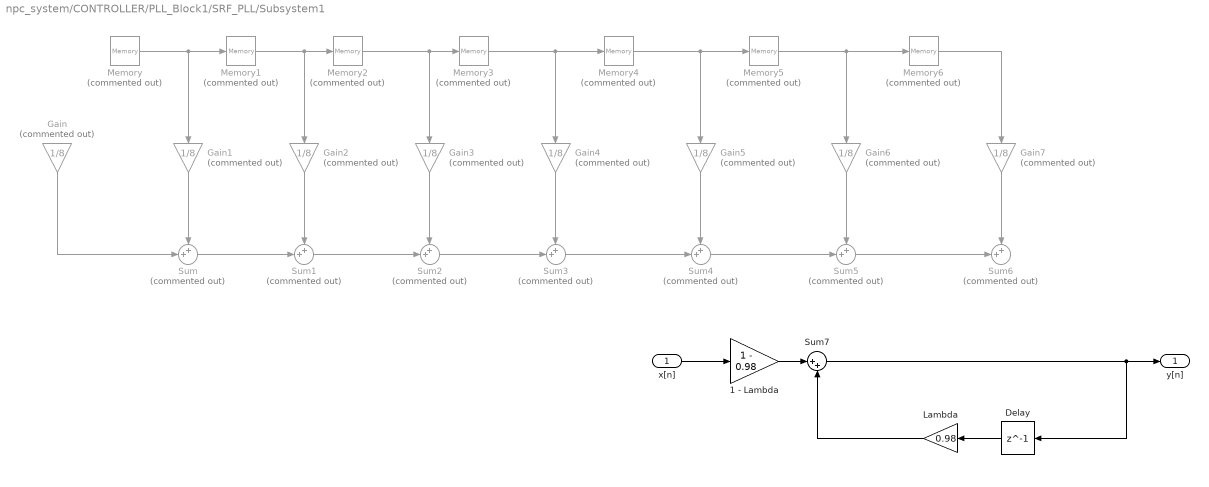
== system npc_system/CONTROLLER/PLL_Block1/SRF_PLL/Subsystem1 ==
  x[n] : Inport
  1 - Lambda : Gain  Gain=1 - 0.98
  Delay : Delay  DelayLength=1
  Gain{,1..7} (8 alike) : Gain  Commented=on  Gain=1/8
  Lambda : Gain  Gain=0.98
  Memory{,1..6} (7 alike) : Memory  Commented=on  InheritSampleTime=on
  Sum{,1..6} (7 alike) : Sum  Commented=on  Inputs=++|
  Sum7 : Sum  Inputs=|++
  y[n] : Outport
  wires:
  Sum7/1 -> y[n]/1, Delay/1
  Delay/1 -> Lambda/1
  1 - Lambda/1 -> Sum7/1
  x[n]/1 -> 1 - Lambda/1
  Lambda/1 -> Sum7/2
  Gain7/1 -> Sum6/1
  Sum5/1 -> Sum6/2
  Memory6/1 -> Gain7/1
  Memory5/1 -> Gain6/1, Memory6/1
  Sum4/1 -> Sum5/2
  Gain6/1 -> Sum5/1
  Gain5/1 -> Sum4/1
  Sum3/1 -> Sum4/2
  Memory4/1 -> Gain5/1, Memory5/1
  Memory3/1 -> Gain4/1, Memory4/1
  Sum2/1 -> Sum3/2
  Gain4/1 -> Sum3/1
  Gain3/1 -> Sum2/1
  Sum1/1 -> Sum2/2
  Gain2/1 -> Sum1/1
  Sum/1 -> Sum1/2
  Gain1/1 -> Sum/1
  Gain/1 -> Sum/2
  Memory2/1 -> Gain3/1, Memory3/1
  Memory1/1 -> Gain2/1, Memory2/1
  Memory/1 -> Gain1/1, Memory1/1

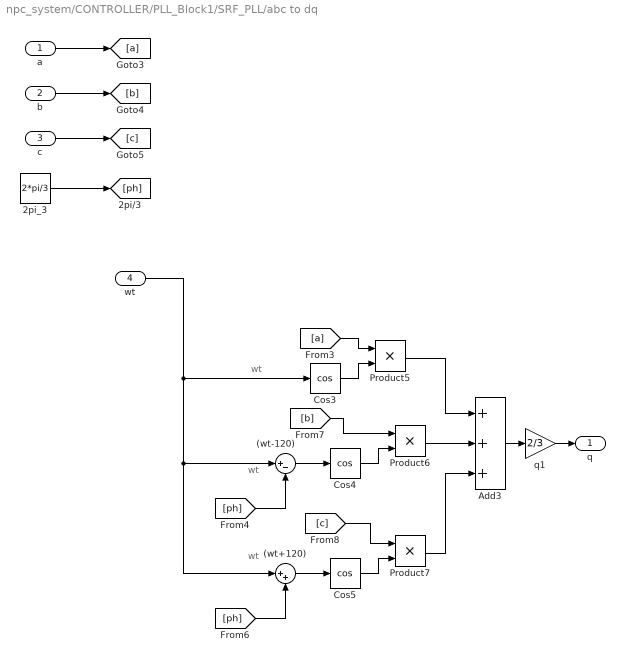
== system npc_system/CONTROLLER/PLL_Block1/SRF_PLL/abc to dq ==
  note: wt
  note: wt
  note: wt
  a : Inport
  b : Inport  Port=2
  c : Inport  Port=3
  wt : Inport  Port=4
  (wt+120) : Sum  Inputs=|++
  (wt-120) : Sum  Inputs=|+-
  2pi_3 : Constant  Value=2*pi/3
  Add3 : Sum  Inputs=+++
  Cos3 : Trigonometry  Operator=cos
  Cos4 : Trigonometry  Operator=cos
  Cos5 : Trigonometry  Operator=cos
  Product5 : Product
  Product6 : Product
  Product7 : Product
  q1 : Gain  Gain=2/3
  q : Outport
  wires:
  [a] -> Product5/1
  Cos3/1 -> Product5/2
  wt/1 -> (wt+120)/1, (wt-120)/1, Cos3/1
  [ph] -> (wt+120)/2
  Product7/1 -> Add3/3
  a/1 -> [a]
  (wt+120)/1 -> Cos5/1
  Product6/1 -> Add3/2
  c/1 -> [c]
  [ph] -> (wt-120)/2
  (wt-120)/1 -> Cos4/1
  [b] -> Product6/1
  Cos4/1 -> Product6/2
  Product5/1 -> Add3/1
  Cos5/1 -> Product7/2
  b/1 -> [b]
  Add3/1 -> q1/1
  [c] -> Product7/1
  q1/1 -> q/1
  2pi_3/1 -> [ph]

== system npc_system/CONTROLLER/PLL_Block1/Subsystem/Initialize at Zero Crossing ==
  In1 : Inport
  Trigger : TriggerPort  VariantControl=Variant
  OR : Logic  Operator=OR  IconShape=distinctive  AllPortsSameDT=off  OutDataTypeStr=boolean
  Unit Delay : UnitDelay  SampleTime=-1  HasFrameUpgradeWarning=on
  Out1 : Outport  InitialOutput=0  VectorParamsAs1DForOutWhenUnconnected=off
  wires:
  OR/1 -> Out1/1, Unit Delay/1
  Unit Delay/1 -> OR/2
  In1/1 -> OR/1

== system npc_system/CONTROLLER/PLL_REF/Subsystem2/Subsystem ==
  u1 : Inport
  Bias : Bias  Bias=-0  SaturateOnIntegerOverflow=off
  Gain : Gain  Gain=1/(2*pi-0)
  Gain1 : Gain  Gain=(2*pi-0)
  Rounding Function : Rounding
  Sum1 : Sum  Inputs=|+-
  y : Outport  VectorParamsAs1DForOutWhenUnconnected=off
  wires:
  Gain1/1 -> Sum1/2
  Bias/1 -> Gain/1
  Sum1/1 -> y/1
  Gain/1 -> Rounding Function/1
  u1/1 -> Bias/1, Sum1/1
  Rounding Function/1 -> Gain1/1

== system npc_system/CONTROLLER/SIM_EPWM_AQ/sim_epwm./codegen ==

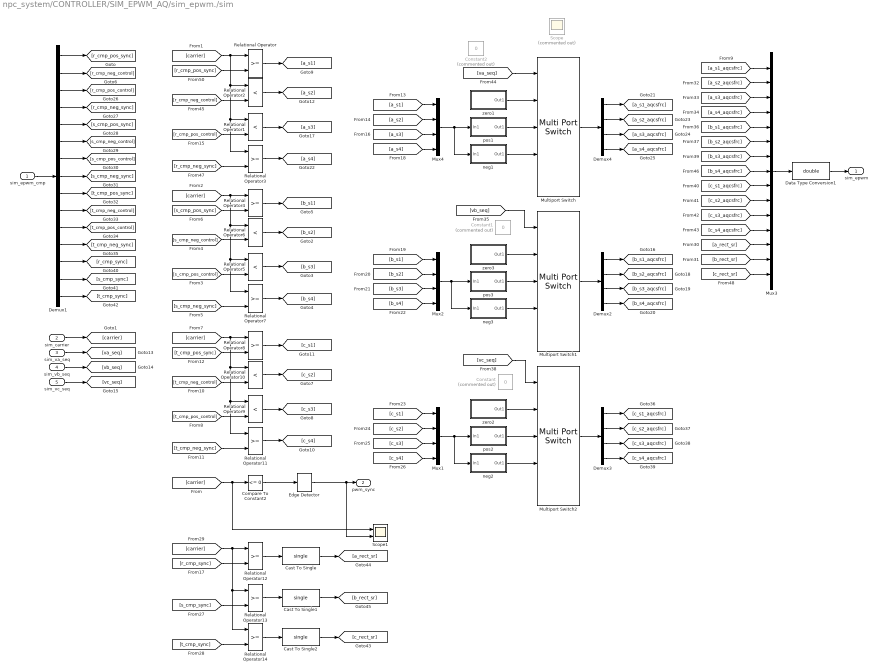
== system npc_system/CONTROLLER/SIM_EPWM_AQ/sim_epwm./sim ==
  sim_epwm_cmp : Inport
  sim_carrier : Inport  Port=2
  sim_va_seq : Inport  Port=3
  sim_vb_seq : Inport  Port=4
  sim_vc_seq : Inport  Port=5
  Cast To Single : DataTypeConversion  OutDataTypeStr=single  SaturateOnIntegerOverflow=off  RndMeth=Floor
  Cast To Single1 : DataTypeConversion  OutDataTypeStr=single  SaturateOnIntegerOverflow=off  RndMeth=Floor
  Cast To Single2 : DataTypeConversion  OutDataTypeStr=single  SaturateOnIntegerOverflow=off  RndMeth=Floor
  Compare To Constant2 : simulink/Logic and Bit Operations/Compare To Constant  relop=<=  const=0  OutDataTypeStr=boolean
  Constant : Constant  Commented=on  Value=0
  Constant1 : Constant  Commented=on  Value=0
  Constant2 : Constant  Commented=on  Value=0
  Data Type Conversion1 : DataTypeConversion  OutDataTypeStr=double  SaturateOnIntegerOverflow=off  RndMeth=Floor
  Demux1 : Demux  Outputs=15
  Demux2 : Demux
  Demux3 : Demux
  Demux4 : Demux
  Edge Detector : spsEdgeDetectorLib/Edge Detector  model=Falling  ic=0  Ts=0
      settings: SourceProductBaseCode=PS
  Multiport Switch : MultiPortSwitch  DataPortOrder=Zero-based contiguous  DataPortForDefault=Additional data port  zeroidx=on  OutDataTypeStr=single  SaturateOnIntegerOverflow=off  InputSameDT=off
  Multiport Switch1 : MultiPortSwitch  DataPortOrder=Zero-based contiguous  DataPortForDefault=Additional data port  zeroidx=on  OutDataTypeStr=single  SaturateOnIntegerOverflow=off  InputSameDT=off
  Multiport Switch2 : MultiPortSwitch  DataPortOrder=Zero-based contiguous  DataPortForDefault=Additional data port  zeroidx=on  OutDataTypeStr=single  SaturateOnIntegerOverflow=off  InputSameDT=off
  Mux1 : Mux
  Mux2 : Mux
  Mux3 : Mux  Inputs=15
  Mux4 : Mux
  Relational Operator{,3..4,7..8,11..14} (9 alike) : RelationalOperator  OutDataTypeStr=boolean  RndMeth=Simplest  InputSameDT=off
  Relational Operator{1..2,5..6,9..10} (6 alike) : RelationalOperator  Operator=<  OutDataTypeStr=boolean  RndMeth=Simplest  InputSameDT=off
  Scope : Scope  Commented=on
  Scope1 : Scope  NumInputPorts=2
  neg1 : Subsystem  TreatAsAtomicUnit=on
      settings: RTWSystemCode=Inline
  neg2 : Subsystem  TreatAsAtomicUnit=on
      settings: RTWSystemCode=Inline
  neg3 : Subsystem  TreatAsAtomicUnit=on
      settings: RTWSystemCode=Inline
  pos1 : Subsystem  TreatAsAtomicUnit=on
      settings: RTWSystemCode=Inline
  pos2 : Subsystem  TreatAsAtomicUnit=on
      settings: RTWSystemCode=Inline
  pos3 : Subsystem  TreatAsAtomicUnit=on
      settings: RTWSystemCode=Inline
  zero1 : Subsystem  TreatAsAtomicUnit=on
      settings: RTWSystemCode=Inline
  zero2 : Subsystem  TreatAsAtomicUnit=on
      settings: RTWSystemCode=Inline
  zero3 : Subsystem  TreatAsAtomicUnit=on
      settings: RTWSystemCode=Inline
  sim_epwm : Outport
  pwm_sync : Outport  Port=2
  wires:
  sim_epwm_cmp/1 -> Demux1/1
  Relational Operator/1 -> [a_s1]
  Relational Operator2/1 -> [a_s2]
  Relational Operator1/1 -> [a_s3]
  [carrier] -> Relational Operator/1, Relational Operator2/1, Relational Operator1/1, Relational Operator3/1
  Relational Operator3/1 -> [a_s4]
  Data Type Conversion1/1 -> sim_epwm/1
  Mux3/1 -> Data Type Conversion1/1
  Demux1/1 -> [r_cmp_pos_sync]
  Demux1/2 -> [r_cmp_neg_control]
  Demux1/3 -> [r_cmp_pos_control]
  Demux1/4 -> [r_cmp_neg_sync]
  Demux1/5 -> [s_cmp_pos_sync]
  Demux1/6 -> [s_cmp_neg_control]
  Demux1/7 -> [s_cmp_pos_control]
  Demux1/8 -> [s_cmp_neg_sync]
  Demux1/9 -> [t_cmp_pos_sync]
  Demux1/10 -> [t_cmp_neg_control]
  Demux1/11 -> [t_cmp_pos_control]
  Demux1/12 -> [t_cmp_neg_sync]
  sim_carrier/1 -> [carrier]
  [carrier] -> Compare To Constant2/1, Scope1/1
  [r_cmp_pos_sync] -> Relational Operator/2
  [r_cmp_neg_control] -> Relational Operator2/2
  [r_cmp_neg_sync] -> Relational Operator3/2
  [r_cmp_pos_control] -> Relational Operator1/2
  [s_cmp_pos_control] -> Relational Operator5/2
  [s_cmp_neg_sync] -> Relational Operator7/2
  [s_cmp_neg_control] -> Relational Operator6/2
  [s_cmp_pos_sync] -> Relational Operator4/2
  Relational Operator7/1 -> [b_s4]
  [carrier] -> Relational Operator7/1, Relational Operator5/1, Relational Operator6/1, Relational Operator4/1
  Relational Operator5/1 -> [b_s3]
  Relational Operator6/1 -> [b_s2]
  Relational Operator4/1 -> [b_s1]
  Relational Operator8/1 -> [c_s1]
  Relational Operator10/1 -> [c_s2]
  Relational Operator9/1 -> [c_s3]
  [carrier] -> Relational Operator8/1, Relational Operator10/1, Relational Operator9/1, Relational Operator11/1
  Relational Operator11/1 -> [c_s4]
  [t_cmp_pos_sync] -> Relational Operator8/2
  [t_cmp_neg_control] -> Relational Operator10/2
  [t_cmp_neg_sync] -> Relational Operator11/2
  [t_cmp_pos_control] -> Relational Operator9/2
  sim_va_seq/1 -> [va_seq]
  sim_vb_seq/1 -> [vb_seq]
  sim_vc_seq/1 -> [vc_seq]
  pos3/1(Out1) -> Multiport Switch1/3
  Demux3/1 -> [c_s1_aqcsfrc]
  [b_s2] -> Mux2/2
  [c_s2] -> Mux1/2
  Demux3/4 -> [c_s4_aqcsfrc]
  Demux2/3 -> [b_s3_aqcsfrc]
  Demux4/3 -> [a_s3_aqcsfrc]
  [b_s4] -> Mux2/4
  Demux2/2 -> [b_s2_aqcsfrc]
  neg2/1(Out1) -> Multiport Switch2/4
  Mux4/1 -> pos1/1(In1), neg1/1(In1)
  Demux4/4 -> [a_s4_aqcsfrc]
  pos1/1(Out1) -> Multiport Switch/3
  neg3/1(Out1) -> Multiport Switch1/4
  zero3/1(Out1) -> Multiport Switch1/2
  Demux3/3 -> [c_s3_aqcsfrc]
  neg1/1(Out1) -> Multiport Switch/4
  Multiport Switch/1 -> Demux4/1
  [a_s1] -> Mux4/1
  [vc_seq] -> Multiport Switch2/1
  [c_s3] -> Mux1/3
  [a_s3] -> Mux4/3
  zero1/1(Out1) -> Multiport Switch/2
  Demux4/2 -> [a_s2_aqcsfrc]
  Demux4/1 -> [a_s1_aqcsfrc]
  Mux1/1 -> neg2/1(In1), pos2/1(In1)
  [b_s1] -> Mux2/1
  [c_s1] -> Mux1/1
  pos2/1(Out1) -> Multiport Switch2/3
  Demux3/2 -> [c_s2_aqcsfrc]
  Multiport Switch1/1 -> Demux2/1
  Mux2/1 -> pos3/1(In1), neg3/1(In1)
  Demux2/1 -> [b_s1_aqcsfrc]
  Multiport Switch2/1 -> Demux3/1
  [c_s4] -> Mux1/4
  [a_s2] -> Mux4/2
  zero2/1(Out1) -> Multiport Switch2/2
  [a_s4] -> Mux4/4
  Demux2/4 -> [b_s4_aqcsfrc]
  [a_s1_aqcsfrc] -> Mux3/1
  [a_s4_aqcsfrc] -> Mux3/4
  [a_s3_aqcsfrc] -> Mux3/3
  [a_s2_aqcsfrc] -> Mux3/2
  [b_s3] -> Mux2/3
  [b_s1_aqcsfrc] -> Mux3/5
  [b_s2_aqcsfrc] -> Mux3/6
  [b_s3_aqcsfrc] -> Mux3/7
  [b_s4_aqcsfrc] -> Mux3/8
  [c_s1_aqcsfrc] -> Mux3/9
  [c_s2_aqcsfrc] -> Mux3/10
  [c_s3_aqcsfrc] -> Mux3/11
  [c_s4_aqcsfrc] -> Mux3/12
  Compare To Constant2/1 -> Edge Detector/1
  Edge Detector/1 -> pwm_sync/1, Scope1/2
  [vb_seq] -> Multiport Switch1/1
  [va_seq] -> Multiport Switch/1
  ? -> Scope/1
  Demux1/13 -> [r_cmp_sync]
  Demux1/14 -> [s_cmp_sync]
  Demux1/15 -> [t_cmp_sync]
  [carrier] -> Relational Operator14/1, Relational Operator13/1, Relational Operator12/1
  [r_cmp_sync] -> Relational Operator12/2
  [s_cmp_sync] -> Relational Operator13/2
  [t_cmp_sync] -> Relational Operator14/2
  Relational Operator14/1 -> Cast To Single2/1
  Relational Operator13/1 -> Cast To Single1/1
  Relational Operator12/1 -> Cast To Single/1
  [a_rect_sr] -> Mux3/13
  [b_rect_sr] -> Mux3/14
  [c_rect_sr] -> Mux3/15
  Cast To Single/1 -> [a_rect_sr]
  Cast To Single1/1 -> [b_rect_sr]
  Cast To Single2/1 -> [c_rect_sr]

== system npc_system/CONTROLLER/PLL_Block1/SRF_PLL/Integrator/Accumulation ==
  In1 : Inport  OutDataTypeStr=single
  Action Port : ActionPort
  Out : Outport  OutDataTypeStr=single
  wires:
  In1/1 -> Out/1

== system npc_system/CONTROLLER/PLL_Block1/SRF_PLL/Integrator/Reset Integrator ==
  Action Port : ActionPort
  Constant1 : Constant  Value=0  OutDataTypeStr=single
  Out : Outport
  wires:
  Constant1/1 -> Out/1

== system npc_system/CONTROLLER/SIM_EPWM_AQ/sim_epwm./sim/neg1 ==
  In1 : Inport
  Constant : Constant  Value=0  OutDataTypeStr=boolean  SampleTime=-1
  Constant1 : Constant  OutDataTypeStr=boolean  SampleTime=-1
  Demux : Demux
  Mux1 : Mux
  Out1 : Outport
  wires:
  In1/1 -> Demux/1
  Mux1/1 -> Out1/1
  Constant/1 -> Mux1/1
  Constant1/1 -> Mux1/3
  Demux/2 -> Mux1/2
  Demux/4 -> Mux1/4

== system npc_system/CONTROLLER/SIM_EPWM_AQ/sim_epwm./sim/neg2 ==
  In1 : Inport
  Constant : Constant  Value=0  OutDataTypeStr=boolean  SampleTime=-1
  Constant1 : Constant  OutDataTypeStr=boolean  SampleTime=-1
  Constant2 : Constant  Value=0  OutDataTypeStr=boolean  SampleTime=-1
  Demux : Demux
  Mux1 : Mux
  Out1 : Outport
  wires:
  In1/1 -> Demux/1
  Mux1/1 -> Out1/1
  Constant/1 -> Mux1/1
  Constant1/1 -> Mux1/3
  Demux/2 -> Mux1/2
  Constant2/1 -> Mux1/4

== system npc_system/CONTROLLER/SIM_EPWM_AQ/sim_epwm./sim/neg3 ==
  In1 : Inport
  Constant : Constant  Value=0  OutDataTypeStr=boolean  SampleTime=-1
  Constant1 : Constant  OutDataTypeStr=boolean  SampleTime=-1
  Constant2 : Constant  Value=0  OutDataTypeStr=boolean  SampleTime=-1
  Demux : Demux
  Mux1 : Mux
  Out1 : Outport
  wires:
  In1/1 -> Demux/1
  Mux1/1 -> Out1/1
  Constant/1 -> Mux1/1
  Constant1/1 -> Mux1/3
  Demux/2 -> Mux1/2
  Constant2/1 -> Mux1/4

== system npc_system/CONTROLLER/SIM_EPWM_AQ/sim_epwm./sim/pos1 ==
  In1 : Inport
  Constant : Constant  Value=0  OutDataTypeStr=boolean  SampleTime=-1
  Constant1 : Constant  OutDataTypeStr=boolean  SampleTime=-1
  Demux : Demux
  Mux1 : Mux
  Out1 : Outport
  wires:
  In1/1 -> Demux/1
  Mux1/1 -> Out1/1
  Constant/1 -> Mux1/4
  Constant1/1 -> Mux1/2
  Demux/3 -> Mux1/3
  Demux/1 -> Mux1/1

== system npc_system/CONTROLLER/SIM_EPWM_AQ/sim_epwm./sim/pos2 ==
  In1 : Inport
  Constant : Constant  Value=0  OutDataTypeStr=boolean  SampleTime=-1
  Constant1 : Constant  OutDataTypeStr=boolean  SampleTime=-1
  Constant2 : Constant  Value=0  OutDataTypeStr=boolean  SampleTime=-1
  Demux : Demux
  Mux1 : Mux
  Out1 : Outport
  wires:
  In1/1 -> Demux/1
  Mux1/1 -> Out1/1
  Constant/1 -> Mux1/4
  Constant1/1 -> Mux1/2
  Demux/3 -> Mux1/3
  Constant2/1 -> Mux1/1

== system npc_system/CONTROLLER/SIM_EPWM_AQ/sim_epwm./sim/pos3 ==
  In1 : Inport
  Constant : Constant  Value=0  OutDataTypeStr=boolean  SampleTime=-1
  Constant1 : Constant  OutDataTypeStr=boolean  SampleTime=-1
  Constant2 : Constant  Value=0  OutDataTypeStr=boolean  SampleTime=-1
  Demux : Demux
  Mux1 : Mux
  Out1 : Outport
  wires:
  In1/1 -> Demux/1
  Mux1/1 -> Out1/1
  Constant/1 -> Mux1/4
  Constant1/1 -> Mux1/2
  Demux/3 -> Mux1/3
  Constant2/1 -> Mux1/1

== system npc_system/CONTROLLER/SIM_EPWM_AQ/sim_epwm./sim/zero1 ==
  Constant{,1..3} (4 alike) : Constant  Value=0  OutDataTypeStr=boolean  SampleTime=-1
  Mux1 : Mux
  Out1 : Outport
  wires:
  Mux1/1 -> Out1/1
  Constant/1 -> Mux1/1
  Constant3/1 -> Mux1/4
  Constant2/1 -> Mux1/3
  Constant1/1 -> Mux1/2

== system npc_system/CONTROLLER/SIM_EPWM_AQ/sim_epwm./sim/zero2 ==
  Constant{,1..3} (4 alike) : Constant  Value=0  OutDataTypeStr=boolean  SampleTime=-1
  Mux1 : Mux
  Out1 : Outport
  wires:
  Mux1/1 -> Out1/1
  Constant/1 -> Mux1/1
  Constant3/1 -> Mux1/4
  Constant2/1 -> Mux1/3
  Constant1/1 -> Mux1/2

== system npc_system/CONTROLLER/SIM_EPWM_AQ/sim_epwm./sim/zero3 ==
  Constant{,1..3} (4 alike) : Constant  Value=0  OutDataTypeStr=boolean  SampleTime=-1
  Mux1 : Mux
  Out1 : Outport
  wires:
  Mux1/1 -> Out1/1
  Constant/1 -> Mux1/1
  Constant3/1 -> Mux1/4
  Constant2/1 -> Mux1/3
  Constant1/1 -> Mux1/2

== stateflow chart npc_system/CONTROLLER/SIM_CMPSS+CLB/SIM_CLB_TILE0 ==
  (default) -> (junction 64)
  (junction 64) -> (junction 67) [order 1] : [cmpssh==double(1) & pwm_sr==double(1)]
  (junction 64) -> (junction 68) [order 2] : {pwm_sr_pos = double(0);}
  (junction 67) -> (junction 70) : {pwm_sr_pos = double(1);}
  (junction 70) -> (junction 68)
  (junction 68) -> (junction 89)
  (junction 89) -> (junction 91) [order 1] : [cmpssl==double(0) & pwm_sr==double(1)]
  (junction 89) -> (junction 86) [order 2] : {pwm_sr_neg = double(0);}
  (junction 91) -> (junction 92) : {pwm_sr_neg = double(1);}
  (junction 86) -> (junction 92)
  data: cmpssh input double; pwm_sr_pos output double; pwm_sr_neg output double; cmpssl input; pwm_sr input double

== stateflow chart npc_system/CONTROLLER/SIM_ADC/Chart2 ==
  state ADCA [parallel]
    settings: executionOrder=1
    state FUNCTION_CALL
      en:
      adcinta;
    (default) -> FUNCTION_CALL
    FUNCTION_CALL -> FUNCTION_CALL
  events: adcinta output FUNCTION_CALL_EVENT

== stateflow chart npc_system/CONTROLLER/SIM_CMPSS+CLB/SIM_CLB_TILE1 ==
  (default) -> (junction 64)
  (junction 64) -> (junction 67) [order 1] : [cmpssh==double(1) & pwm_sr==double(1)]
  (junction 64) -> (junction 68) [order 2] : {pwm_sr_pos = double(0);}
  (junction 67) -> (junction 70) : {pwm_sr_pos = double(1);}
  (junction 70) -> (junction 68)
  (junction 68) -> (junction 89)
  (junction 89) -> (junction 91) [order 1] : [cmpssl==double(0) & pwm_sr==double(1)]
  (junction 89) -> (junction 86) [order 2] : {pwm_sr_neg = double(0);}
  (junction 91) -> (junction 92) : {pwm_sr_neg = double(1);}
  (junction 86) -> (junction 92)
  data: cmpssh input double; pwm_sr_pos output double; pwm_sr_neg output double; cmpssl input; pwm_sr input double

== stateflow chart npc_system/CONTROLLER/SIM_CMPSS+CLB/SIM_CLB_TILE2 ==
  (default) -> (junction 64)
  (junction 64) -> (junction 67) [order 1] : [cmpssh==double(1) & pwm_sr==double(1)]
  (junction 64) -> (junction 68) [order 2] : {pwm_sr_pos = double(0);}
  (junction 67) -> (junction 70) : {pwm_sr_pos = double(1);}
  (junction 70) -> (junction 68)
  (junction 68) -> (junction 89)
  (junction 89) -> (junction 91) [order 1] : [cmpssl==double(0) & pwm_sr==double(1)]
  (junction 89) -> (junction 86) [order 2] : {pwm_sr_neg = double(0);}
  (junction 91) -> (junction 92) : {pwm_sr_neg = double(1);}
  (junction 86) -> (junction 92)
  data: cmpssh input double; pwm_sr_pos output double; pwm_sr_neg output double; cmpssl input; pwm_sr input double

== stateflow chart npc_system/CONTROLLER/SIM_CMPSS+CLB/SIM_CMPSS4 ==
  (default) -> (junction 15) [commented out]
  (default) -> (junction 56)
  (junction 15) -> (junction 17) [commented out] : [iL>uint16(2171)]
  (junction 15) -> (junction 19) [commented out]
  (junction 17) -> (junction 29) [commented out] : {
      | cmpssh = uint16(1);
      | cmpssl = uint16(0);
      | }
  (junction 56) -> (junction 44) [order 1] : [iL>uint16(2171)]
  (junction 56) -> (junction 49) [order 2] : {cmpssh = uint16(0);}
  (junction 44) -> (junction 55) : {cmpssh = uint16(1);}
  (junction 19) -> (junction 21) [commented out] : [iL<uint16(1923)]
  (junction 19) -> (junction 24) [commented out] : {
      | cmpssh = uint16(0);
      | cmpssl = uint16(0);
      | }
  (junction 21) -> (junction 25) [commented out] : {
      | cmpssh = uint16(0);
      | cmpssl = uint16(1);
      | }
  (junction 55) -> (junction 49)
  (junction 49) -> (junction 58)
  (junction 24) -> (junction 25) [commented out]
  (junction 25) -> (junction 29) [commented out]
  (junction 58) -> (junction 65) [order 1] : [iL>uint16(1923)]
  (junction 58) -> (junction 61) [order 2] : {cmpssl = uint16(0);}
  (junction 65) -> (junction 60) : {cmpssl = uint16(1);}
  (junction 61) -> (junction 60)
  data: iL input double; cmpssh output double; cmpssl output double

== stateflow chart npc_system/CONTROLLER/SIM_CMPSS+CLB/SIM_CMPSS1 ==
  (default) -> (junction 15) [commented out]
  (default) -> (junction 56)
  (junction 15) -> (junction 17) [commented out] : [iL>uint16(2171)]
  (junction 15) -> (junction 19) [commented out]
  (junction 17) -> (junction 29) [commented out] : {
      | cmpssh = uint16(1);
      | cmpssl = uint16(0);
      | }
  (junction 56) -> (junction 44) [order 1] : [iL>uint16(2171)]
  (junction 56) -> (junction 49) [order 2] : {cmpssh = uint16(0);}
  (junction 44) -> (junction 55) : {cmpssh = uint16(1);}
  (junction 19) -> (junction 21) [commented out] : [iL<uint16(1923)]
  (junction 19) -> (junction 24) [commented out] : {
      | cmpssh = uint16(0);
      | cmpssl = uint16(0);
      | }
  (junction 21) -> (junction 25) [commented out] : {
      | cmpssh = uint16(0);
      | cmpssl = uint16(1);
      | }
  (junction 55) -> (junction 49)
  (junction 49) -> (junction 58)
  (junction 24) -> (junction 25) [commented out]
  (junction 25) -> (junction 29) [commented out]
  (junction 58) -> (junction 65) [order 1] : [iL>uint16(1923)]
  (junction 58) -> (junction 61) [order 2] : {cmpssl = uint16(0);}
  (junction 65) -> (junction 60) : {cmpssl = uint16(1);}
  (junction 61) -> (junction 60)
  data: iL input double; cmpssh output double; cmpssl output double

== stateflow chart npc_system/CONTROLLER/SIM_CMPSS+CLB/SIM_CMPSS2 ==
  (default) -> (junction 15) [commented out]
  (default) -> (junction 56)
  (junction 15) -> (junction 17) [commented out] : [iL>uint16(2171)]
  (junction 15) -> (junction 19) [commented out]
  (junction 17) -> (junction 29) [commented out] : {
      | cmpssh = uint16(1);
      | cmpssl = uint16(0);
      | }
  (junction 56) -> (junction 44) [order 1] : [iL>uint16(2171)]
  (junction 56) -> (junction 49) [order 2] : {cmpssh = uint16(0);}
  (junction 44) -> (junction 55) : {cmpssh = uint16(1);}
  (junction 19) -> (junction 21) [commented out] : [iL<uint16(1923)]
  (junction 19) -> (junction 24) [commented out] : {
      | cmpssh = uint16(0);
      | cmpssl = uint16(0);
      | }
  (junction 21) -> (junction 25) [commented out] : {
      | cmpssh = uint16(0);
      | cmpssl = uint16(1);
      | }
  (junction 55) -> (junction 49)
  (junction 49) -> (junction 58)
  (junction 24) -> (junction 25) [commented out]
  (junction 25) -> (junction 29) [commented out]
  (junction 58) -> (junction 65) [order 1] : [iL>uint16(1923)]
  (junction 58) -> (junction 61) [order 2] : {cmpssl = uint16(0);}
  (junction 65) -> (junction 60) : {cmpssl = uint16(1);}
  (junction 61) -> (junction 60)
  data: iL input double; cmpssh output double; cmpssl output double
